simulink library "HEV_lib"  (Simulink 7.7)
settings: Solver=ode45  SolverMode=SingleTasking  StartTime=0.0  StopTime=10.0  RelTol=1e-3
undefined symbols (not defined in the file): DiscIntNeverNeededParam, Hydride, magnitude, Metal, Nickel, Ts
libraries: powerlib x72, driveline x12, simulink_extras x8, electricdrivelib x7, simulink x6, powerlib_extras x2, HEV_lib x1
(part 3 of 3)

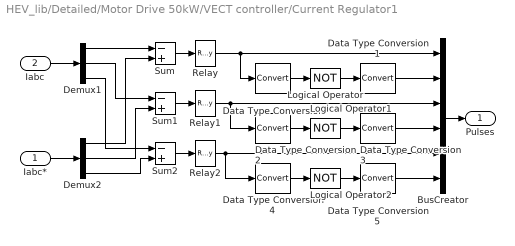
== system HEV_lib/Detailed/Motor Drive 50kW/VECT controller/Current Regulator1 ==
  Iabc* : Inport
  Iabc : Inport  Port=2
  BusCreator : BusCreator  Inputs=6
  Data Type Conversion{,1..5} (6 alike) : DataTypeConversion  SaturateOnIntegerOverflow=on  RndMeth=Zero
  Demux1 : Demux  Outputs=3
  Demux2 : Demux  Outputs=3
  Logical Operator : Logic  Operator=NOT
  Logical Operator1 : Logic  Operator=NOT
  Logical Operator2 : Logic  Operator=NOT
  Relay : Relay  OnSwitchValue=h/2  OffSwitchValue=-h/2
  Relay1 : Relay  OnSwitchValue=h/2  OffSwitchValue=-h/2
  Relay2 : Relay  OnSwitchValue=h/2  OffSwitchValue=-h/2
  Sum : Sum  Inputs=-+  SaturateOnIntegerOverflow=on  InputSameDT=on  OutDataTypeStr=Inherit: Same as first input
  Sum1 : Sum  Inputs=-+  SaturateOnIntegerOverflow=on  InputSameDT=on  OutDataTypeStr=Inherit: Same as first input
  Sum2 : Sum  Inputs=-+  SaturateOnIntegerOverflow=on  InputSameDT=on  OutDataTypeStr=Inherit: Same as first input
  Pulses : Outport  InitialOutput=0
  wires:
  Data Type Conversion5/1 -> BusCreator/6
  Data Type Conversion4/1 -> Logical Operator2/1
  Data Type Conversion3/1 -> BusCreator/4
  Data Type Conversion2/1 -> Logical Operator1/1
  Data Type Conversion1/1 -> BusCreator/2
  Data Type Conversion/1 -> Logical Operator/1
  Sum/1 -> Relay/1
  Sum1/1 -> Relay1/1
  Demux1/1 -> Sum/1
  Demux1/2 -> Sum1/1
  BusCreator/1 -> Pulses/1
  Iabc/1 -> Demux1/1
  Sum2/1 -> Relay2/1
  Demux1/3 -> Sum2/1
  Demux2/3 -> Sum2/2
  Demux2/2 -> Sum1/2
  Demux2/1 -> Sum/2
  Iabc*/1 -> Demux2/1
  Relay/1 -> Data Type Conversion/1, BusCreator/1
  Relay1/1 -> Data Type Conversion2/1, BusCreator/3
  Relay2/1 -> Data Type Conversion4/1, BusCreator/5
  Logical Operator/1 -> Data Type Conversion1/1
  Logical Operator1/1 -> Data Type Conversion3/1
  Logical Operator2/1 -> Data Type Conversion5/1

== system HEV_lib/Detailed/Motor Drive 50kW/VECT controller/DQ-ABC ==
  "Iq* " : Inport
  "Id* " : Inport  Port=2
  Teta : Inport  Port=3
  Fcn : Fcn  Expr=sin(u)
  Fcn1 : Fcn  Expr=cos(u)
  Gain2 : Gain  SaturateOnIntegerOverflow=on  OutDataTypeStr=Inherit: Same as input  ParamDataTypeStr=Inherit: Same as input
  Gain3 : Gain  SaturateOnIntegerOverflow=on  OutDataTypeStr=Inherit: Same as input  ParamDataTypeStr=Inherit: Same as input
  Gain4 : Gain  SaturateOnIntegerOverflow=on  OutDataTypeStr=Inherit: Same as input  ParamDataTypeStr=Inherit: Same as input
  Mux : Mux
  Mux2 : Mux  Inputs=3
  ia : Fcn  Expr=-u[3]*u[2] + u[4]*u[1]
  ib : Fcn  Expr=(-u[1]+1.7320508*u[2])*u[4]*0.5+(u[2]+1.7320508*u[1])*u[3]*0.5
  ic : Sum  Inputs=--  SaturateOnIntegerOverflow=on  InputSameDT=on  OutDataTypeStr=Inherit: Same as first input
  Iabc* : Outport  InitialOutput=0
  wires:
  ib/1 -> ic/1, Gain3/1
  ia/1 -> ic/2, Gain2/1
  Gain2/1 -> Mux2/1
  Gain4/1 -> Mux2/3
  ic/1 -> Gain4/1
  Gain3/1 -> Mux2/2
  "Iq* "/1 -> Mux/4
  "Id* "/1 -> Mux/3
  Teta/1 -> Fcn/1, Fcn1/1
  Mux/1 -> ia/1, ib/1
  Mux2/1 -> Iabc*/1
  Fcn1/1 -> Mux/1
  Fcn/1 -> Mux/2

== system HEV_lib/Average-values/Generator Drive 30kW/Three-phase Inverter/Id computation/Demux ==
  m : Inport
  Demux1 : Demux  Outputs=5
  Terminator : Terminator
  Vac : Outport
  Ia : Outport  Port=2
  Vbc : Outport  Port=3
  Ib : Outport  Port=4
  wires:
  Demux1/3 -> Terminator/1  "Ic"
  Demux1/1 -> Ia/1  "Ia"
  Demux1/2 -> Ib/1  "Ib"
  Demux1/4 -> Vac/1  "Vac"
  Demux1/5 -> Vbc/1  "Vbc"
  m/1 -> Demux1/1

== system HEV_lib/Average-values/Generator Drive 30kW/Three-phase Inverter/Id computation/Demux1 ==
  m : Inport
  Demux1 : Demux  Outputs=5
  Terminator1 : Terminator
  Terminator2 : Terminator
  Ia : Outport
  Ib : Outport  Port=2
  Ic : Outport  Port=3
  wires:
  m/1 -> Demux1/1
  Demux1/5 -> Terminator2/1  "Vbc"
  Demux1/4 -> Terminator1/1  "Vac"
  Demux1/2 -> Ib/1  "Ib"
  Demux1/1 -> Ia/1  "Ia"
  Demux1/3 -> Ic/1  "Ic"

== system HEV_lib/Average-values/Motor Drive 50kW/Three-phase Inverter/Id computation/Demux ==
  m : Inport
  Demux1 : Demux  Outputs=5
  Terminator : Terminator
  Vac : Outport
  Ia : Outport  Port=2
  Vbc : Outport  Port=3
  Ib : Outport  Port=4
  wires:
  m/1 -> Demux1/1
  Demux1/5 -> Vbc/1  "Vbc"
  Demux1/4 -> Vac/1  "Vac"
  Demux1/2 -> Ib/1  "Ib"
  Demux1/1 -> Ia/1  "Ia"
  Demux1/3 -> Terminator/1  "Ic"

== system HEV_lib/Average-values/Motor Drive 50kW/Three-phase Inverter/Id computation/Demux1 ==
  m : Inport
  Demux1 : Demux  Outputs=5
  Terminator1 : Terminator
  Terminator2 : Terminator
  Ia : Outport
  Ib : Outport  Port=2
  Ic : Outport  Port=3
  wires:
  Demux1/3 -> Ic/1  "Ic"
  Demux1/1 -> Ia/1  "Ia"
  Demux1/2 -> Ib/1  "Ib"
  Demux1/4 -> Terminator1/1  "Vac"
  Demux1/5 -> Terminator2/1  "Vbc"
  m/1 -> Demux1/1

== matlab function Average-values/Motor Drive 50kW/VECT controller/MTPA Field Weakening Controller ==
  data: iqn_opt input double; Ten input double; iqn output double; w input double; Vdc input double; params input double; idn output double
function [iqn,idn] = fcn(iqn_opt,Ten,w,Vdc,params)
% Maximum Torque Per Ampere (MTPA) Field Weakening Controller

kFact = 0.9;
Ld = params(1);
Lq = params(2);
lam = params(3);
p = params(4);
ib = params(5);
Vs = Vdc/(pi/2)*kFact;
ten = abs(Ten);
iqn = sign(Ten)*iqn_opt;
if Ten == 0 && w == 0
    idn = 0;
elseif iqn == 0
    idn = -(lam*p*w-Vs*kFact)/(p*Ld*w*ib);
else
    idn = 1-Ten/iqn;
end
if sqrt((-Lq*p*w*iqn*ib)^2+(Ld*p*w*idn*ib+lam*p*w)^2) >= Vs 
    vs = Vs;
    k1 = 2*lam*Ld/(ib*Lq^2);
    k2 = Ld^2/Lq^2;
    k3 = lam^2/(ib^2*Lq^2)+k2;
    
    g2 = -vs^2/(p^2*ib^2*Lq^2*w^2) + k1 + k3;
    g3 = -k1*ten-2*ten*k2;
    g4 = k2*ten^2;
    
    a1 = abs(-768*g4^3+384*g4^2*g2^2-48*g4*g2^4-432*g2*g4*g3^2+81*g3^4+12*g3^2*g2^3)^(1/2);
    a2 = (-288*g2*g4+108*g3^2+8*g2^3+12*a1)^(1/3);
    a3 = (-4*g2+a2+48/a2*g4+4/a2*g2^2)^(1/2);
    iqn = (1/12*6^(1/2)*a3+1/12*abs(-48*g2-6*a2-288/a2*g4-24/a2*g2^2-72/a3*g3*6^(1/2))^(1/2));
    iqn = sign(Ten)*iqn;

    idn = 1-Ten/iqn;
end

== matlab function Detailed/Motor Drive 50kW/VECT controller/MTPA Field Weakening Controller ==
  data: iqn_opt input double; Ten input double; iqn output double; w input double; Vdc input double; params input double; idn output double
function [iqn,idn] = fcn(iqn_opt,Ten,w,Vdc,params)
% Maximum Torque Per Ampere (MTPA) Field Weakening Controller

kFact = 0.9;
Ld = params(1);
Lq = params(2);
lam = params(3);
p = params(4);
ib = params(5);
Vs = Vdc/(pi/2)*kFact;
ten = abs(Ten);
iqn = sign(Ten)*iqn_opt;
if Ten == 0 && w == 0
    idn = 0;
elseif iqn == 0
    idn = -(lam*p*w-Vs*kFact)/(p*Ld*w*ib);
else
    idn = 1-Ten/iqn;
end
if sqrt((-Lq*p*w*iqn*ib)^2+(Ld*p*w*idn*ib+lam*p*w)^2) >= Vs 
    vs = Vs;
    k1 = 2*lam*Ld/(ib*Lq^2);
    k2 = Ld^2/Lq^2;
    k3 = lam^2/(ib^2*Lq^2)+k2;
    
    g2 = -vs^2/(p^2*ib^2*Lq^2*w^2) + k1 + k3;
    g3 = -k1*ten-2*ten*k2;
    g4 = k2*ten^2;
    
    a1 = abs(-768*g4^3+384*g4^2*g2^2-48*g4*g2^4-432*g2*g4*g3^2+81*g3^4+12*g3^2*g2^3)^(1/2);
    a2 = (-288*g2*g4+108*g3^2+8*g2^3+12*a1)^(1/3);
    a3 = (-4*g2+a2+48/a2*g4+4/a2*g2^2)^(1/2);
    iqn = (1/12*6^(1/2)*a3+1/12*abs(-48*g2-6*a2-288/a2*g4-24/a2*g2^2-72/a3*g3*6^(1/2))^(1/2));
    iqn = sign(Ten)*iqn;

    idn = 1-Ten/iqn;
end
